simulink model "HANcoder_E407_TTA_CombineModel"  (R2022b)
settings: Solver=FixedStepDiscrete  StartTime=0.0  StopTime=1  FixedStep=0.001  RelTol=1e-3
PreLoadFcn:
  | librarySetup
  | eval([bdroot,'_startup']) %Calling [modelName]_startup.m
values from neighbouring files (symbols this model uses):
  ClockOn = Simulink.Parameter    [HANcoder_E407_TTA_Chris_startup.m]    (also in HANcoder_E407_TTA_CombineModel_Membership_2022a_startup.m; HANcoder_E407_TTA_CombineModel_Membership_startup.m; HANcoder_E407_TTA_CombineModel_V2_startup.m; HANcoder_E407_TTA_CombineModel_startup.m)
  controlWidth = Simulink.Parameter    [HANcoder_E407_TTA_CombineModel_Membership_2022a_startup.m]    (also in HANcoder_E407_TTA_CombineModel_Membership_startup.m; HANcoder_E407_TTA_CombineModel_V2_startup.m; HANcoder_E407_TTA_CombineModel_startup.m)
  desiredAngle = Simulink.Parameter    [HANcoder_E407_TTA_CombineModel_Membership_2022a_startup.m]    (also in HANcoder_E407_TTA_CombineModel_Membership_startup.m; HANcoder_E407_TTA_CombineModel_V2_startup.m; HANcoder_E407_TTA_CombineModel_startup.m)
  frequency_IRQ = 1000    [HANcoder_E407_TTA_Chris_startup.m]    (also in HANcoder_E407_TTA_CombineModel_Membership_2022a_startup.m; HANcoder_E407_TTA_CombineModel_Membership_startup.m; HANcoder_E407_TTA_CombineModel_V2_startup.m; HANcoder_E407_TTA_CombineModel_startup.m)
  intVal = Simulink.Parameter    [HANcoder_E407_TTA_CombineModel_Membership_2022a_startup.m]    (also in HANcoder_E407_TTA_CombineModel_Membership_startup.m; HANcoder_E407_TTA_CombineModel_V2_startup.m; HANcoder_E407_TTA_CombineModel_startup.m)
  L0b = 1    [HANcoder_E407_KinematicAngleControl_startup.m]    (also in HANcoder_E407_TTA_CombineModel_Membership_2022a_startup.m; HANcoder_E407_TTA_CombineModel_Membership_startup.m; HANcoder_E407_TTA_CombineModel_V2_startup.m; HANcoder_E407_TTA_CombineModel_startup.m)
  L0F = 3    [HANcoder_E407_KinematicAngleControl_startup.m]    (also in HANcoder_E407_TTA_CombineModel_Membership_2022a_startup.m; HANcoder_E407_TTA_CombineModel_Membership_startup.m; HANcoder_E407_TTA_CombineModel_V2_startup.m; HANcoder_E407_TTA_CombineModel_startup.m)
  L1F = 4    [HANcoder_E407_KinematicAngleControl_startup.m]    (also in HANcoder_E407_TTA_CombineModel_Membership_2022a_startup.m; HANcoder_E407_TTA_CombineModel_Membership_startup.m; HANcoder_E407_TTA_CombineModel_V2_startup.m; HANcoder_E407_TTA_CombineModel_startup.m)
  matrixRows = Simulink.Parameter    [HANcoder_E407_TTA_Chris_startup.m]    (also in HANcoder_E407_TTA_CombineModel_Membership_2022a_startup.m; HANcoder_E407_TTA_CombineModel_Membership_startup.m; HANcoder_E407_TTA_CombineModel_V2_startup.m; HANcoder_E407_TTA_CombineModel_startup.m)
  MMBS1_ID = Simulink.Parameter    [HANcoder_E407_TTA_Chris_startup.m]    (also in HANcoder_E407_TTA_CombineModel_Membership_2022a_startup.m; HANcoder_E407_TTA_CombineModel_Membership_startup.m; HANcoder_E407_TTA_CombineModel_V2_startup.m; HANcoder_E407_TTA_CombineModel_startup.m)
  propVal = Simulink.Parameter    [HANcoder_E407_TTA_CombineModel_Membership_2022a_startup.m]    (also in HANcoder_E407_TTA_CombineModel_Membership_startup.m; HANcoder_E407_TTA_CombineModel_V2_startup.m; HANcoder_E407_TTA_CombineModel_startup.m)
  ResetPosition = Simulink.Parameter    [HANcoder_E407_TTA_CombineModel_Membership_2022a_startup.m]    (also in HANcoder_E407_TTA_CombineModel_V2_startup.m)
  slotTime = Simulink.Parameter    [HANcoder_E407_TTA_Chris_startup.m]    (also in HANcoder_E407_TTA_CombineModel_Membership_2022a_startup.m; HANcoder_E407_TTA_CombineModel_Membership_startup.m; HANcoder_E407_TTA_CombineModel_V2_startup.m; HANcoder_E407_TTA_CombineModel_startup.m)
  SSTM1_ID = Simulink.Parameter    [HANcoder_E407_TTA_Chris_startup.m]    (also in HANcoder_E407_TTA_CombineModel_Membership_2022a_startup.m; HANcoder_E407_TTA_CombineModel_Membership_startup.m; HANcoder_E407_TTA_CombineModel_V2_startup.m; HANcoder_E407_TTA_CombineModel_startup.m)
  SYNC1_ID = Simulink.Parameter    [HANcoder_E407_TTA_Chris_startup.m]    (also in HANcoder_E407_TTA_CombineModel_Membership_2022a_startup.m; HANcoder_E407_TTA_CombineModel_Membership_startup.m; HANcoder_E407_TTA_CombineModel_V2_startup.m; HANcoder_E407_TTA_CombineModel_startup.m)
  TRCK1_ID1 = Simulink.Parameter    [HANcoder_E407_TTA_Chris_startup.m]    (also in HANcoder_E407_TTA_CombineModel_Membership_2022a_startup.m; HANcoder_E407_TTA_CombineModel_Membership_startup.m; HANcoder_E407_TTA_CombineModel_V2_startup.m; HANcoder_E407_TTA_CombineModel_startup.m)
  TRCK1_ID2 = Simulink.Parameter    [HANcoder_E407_TTA_Chris_startup.m]    (also in HANcoder_E407_TTA_CombineModel_Membership_2022a_startup.m; HANcoder_E407_TTA_CombineModel_Membership_startup.m; HANcoder_E407_TTA_CombineModel_V2_startup.m; HANcoder_E407_TTA_CombineModel_startup.m)
  TRCK1_ID3 = Simulink.Parameter    [HANcoder_E407_TTA_Chris_startup.m]    (also in HANcoder_E407_TTA_CombineModel_Membership_2022a_startup.m; HANcoder_E407_TTA_CombineModel_Membership_startup.m; HANcoder_E407_TTA_CombineModel_V2_startup.m; HANcoder_E407_TTA_CombineModel_startup.m)
  TRLS1_ID4 = Simulink.Parameter    [HANcoder_E407_TTA_Chris_startup.m]    (also in HANcoder_E407_TTA_CombineModel_Membership_2022a_startup.m; HANcoder_E407_TTA_CombineModel_Membership_startup.m; HANcoder_E407_TTA_CombineModel_V2_startup.m; HANcoder_E407_TTA_CombineModel_startup.m)
  TRLS1_ID5 = Simulink.Parameter    [HANcoder_E407_TTA_Chris_startup.m]    (also in HANcoder_E407_TTA_CombineModel_Membership_2022a_startup.m; HANcoder_E407_TTA_CombineModel_Membership_startup.m; HANcoder_E407_TTA_CombineModel_V2_startup.m; HANcoder_E407_TTA_CombineModel_startup.m)
  V2 = 1.3889    [HANcoder_E407_KinematicAngleControl_startup.m]    (also in HANcoder_E407_TTA_CombineModel_Membership_2022a_startup.m = 0.5; HANcoder_E407_TTA_CombineModel_Membership_startup.m = 0.5; HANcoder_E407_TTA_CombineModel_V2_startup.m = 0.5; HANcoder_E407_TTA_CombineModel_startup.m = 0.5)
undefined symbols (not defined in the file or in its folder): A2, A3, A4, CON2, CON3, CON4, D10, D4, D5
libraries: hdlsllib x95, HANcoder_STM32_Target x23, simulink_extras x4, dspstat3 x3, simulink x2, slpidlib x1
(part 1 of 5)
settings Model: Creator=Jason van Kolfschoten  LastModifiedBy=Admin.cvanderspek
settings SolverCC: AlgebraicLoopSolver=TrustRegion  PositivePriorityOrder=on
settings DataIOCC: LimitDataPoints=on  SaveFormat=Array  SignalLoggingSaveFormat=ModelDataLogs  SaveOutput=off  SignalLogging=off  DSMLogging=off  SaveTime=off  ReturnWorkspaceOutputs=off
settings OptimizationCC: BlockReduction=off  DefaultParameterBehavior=Inlined  DefaultUnderspecifiedDataType=single  InlineInvariantSignals=on  ExpressionDepthLimit=2147483647  StateBitsets=on  DataBitsets=on  ZeroExternalMemoryAtStartup=off  ZeroInternalMemoryAtStartup=off  InitFltsAndDblsToZero=on  NoFixptDivByZeroProtection=on  EfficientFloat2IntCast=on  LifeSpan=inf  EfficientTunableParamExpr=on
settings DebuggingCC: SaveWithDisabledLinksMsg=none  SaveWithParameterizedLinksMsg=none  CheckSSInitialOutputMsg=off  UnderspecifiedInitializationDetection=Classic  MergeDetectMultiDrivingBlocksExec=none  SignalResolutionControl=TryResolveAll  SolverPrmCheckMsg=warning  InheritedTsInSrcMsg=none  MultiTaskDSMMsg=warning  MultiTaskCondExecSysMsg=none  ParameterPrecisionLossMsg=none  FcnCallInpInsideContextMsg=warning  UnconnectedInputMsg=warning  UnconnectedOutputMsg=warning  UnconnectedLineMsg=warning  StateNameClashWarn=warning  SFUnexpectedBacktrackingDiag=warning  SFNoUnconditionalDefaultTransitionDiag=warning  SFExecutionAtInitializationDiag=none  SFMachineParentedDataDiag=warning  ArithmeticOperatorsInVariantConditions=warning
settings HardwareCC: ProdBitPerPointer=32  ProdBitPerSizeT=32  ProdBitPerPtrDiffT=32  ProdLargestAtomicInteger=Long  ProdLargestAtomicFloat=Double  ProdWordSize=32  ProdHWDeviceType=ARM Compatible->ARM Cortex  TargetEndianess=LittleEndian  TargetHWDeviceType=Infineon->TriCore
settings ModelReferenceCC: PropagateSignalLabelsOutOfModel=off
settings SFSimCC: SimUseLocalCustomCode=off  MATLABDynamicMemAlloc=off  CustomCodeUndefinedFunction=UseInterfaceOnly
settings RTWCC: Description=Real-Time Workshop Embedded Coder (no auto configuration)  SystemTargetFile=ert.tlc  MakeCommand=make_rtw SHELL= HANcoder_PORTABLE=1 HANcoder_BOOTLOADER=1  TemplateMakefile=STM32_E407_gcc.tmf  RTWUseLocalCustomCode=off
settings CodeAppCC: ForceParamTrailComments=on  IgnoreCustomStorageClasses=off  SimulinkDataObjDesc=on  CustomSymbolStrGlobalVar=rt$N$M  CustomSymbolStrType=$N$M  CustomSymbolStrFcn=$N$M$F  CustomSymbolStrMacro=$N$M  InsertBlockDesc=on  StateflowObjectComments=on  InternalIdentifier=Classic
settings ERTTargetCC: TargetFcnLib=ansi_tfl_tmw.mat  MultiwordLength=2048  IncludeMdlTerminateFcn=off  SuppressErrorStatus=on  SupportNonFinite=off  GenerateASAP2=on  InlinedParameterPlacement=NonHierarchical  ERTCustomFileTemplate=example_file_process.tlc  ConvertIfToSwitch=off  SuppressUnreachableDefaultCases=off
settings ConfigComp: CovMetricSettings=dw  CovSaveCumulativeToWorkspaceVar=on  CovSaveSingleToWorkspaceVar=on  CovExternalEMLEnable=off  CovSFcnEnable=off  DVMaxProcessTime=600  DVAutomaticStubbing=off  DVModelCoverageObjectives=MCDC  DVMaxTestCaseSteps=500  DVTestSuiteOptimization=CombinedObjectives  DVDetectActiveLogic=on  DVSaveHarnessModel=on  DVHarnessSource=Signal Editor

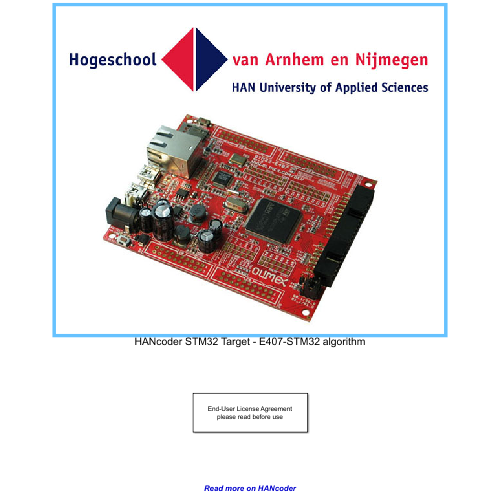
[thumbnail: Simulink's stored preview of the top-level diagram]
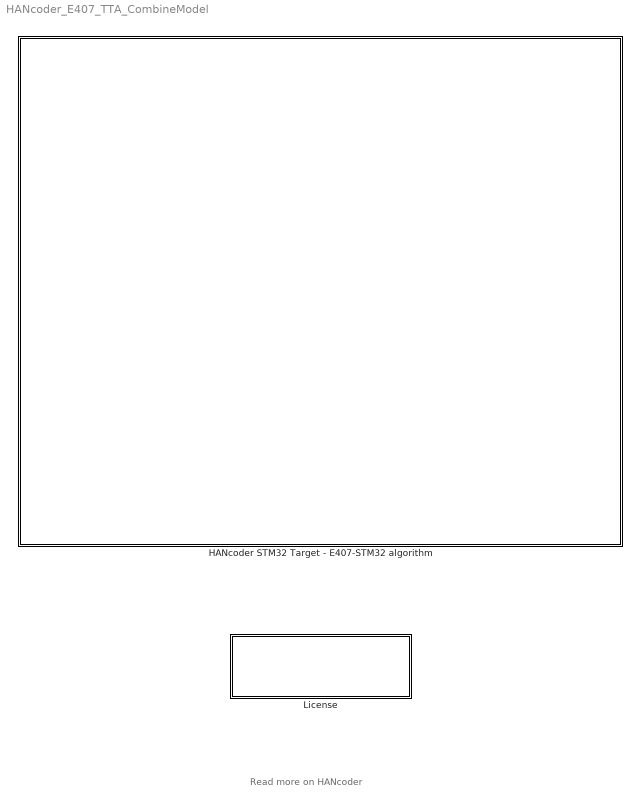
== system HANcoder_E407_TTA_CombineModel ==
  note: Read more on HANcoder
  HANcoder STM32 Target - E407-STM32 algorithm : Subsystem  mask(TopLevelSubsystem){}
      settings: CopyFcn=HANcoderChecks('Copy');  NameChangeFcn=HANcoderChecks('NameChangeE407');  MoveFcn=HANcoderChecks('MoveE407');
      mask Display: image(imread('STM32_E407_HAN.jpg'))
  License : Subsystem  mask(License){}
      settings: NameChangeFcn=HANcoderChecks('NameChangeLicenseBlock');  OpenFcn=winopen('License.pdf')  MoveFcn=HANcoderChecks('MoveLicenseBlock');
      mask Display: disp(['End-User License Agreement\n','please read before use']);

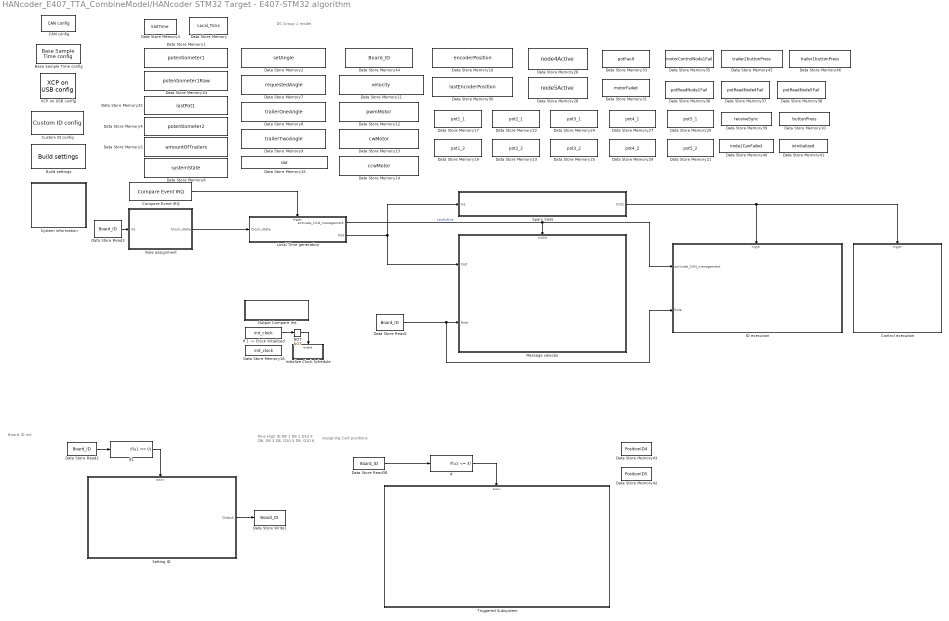
== system HANcoder_E407_TTA_CombineModel/HANcoder STM32 Target - E407-STM32 algorithm ==
  note: DS Group 1 model
  note: Assigning Cart positions
  note: Board ID init
  note: Pins High      		ID
      | D8                 		1
      | D9				2
      | D10				4
      | D8, D9			3
      | D8, D10			5
      | D9, D10			6
  Base Sample Time config : HANcoder_STM32_Target/STM32-E407/System Config/Base Sample Time config  Tag=HANcoder_TARGET_STM32_E407  Description=HANcoder Target STM32-E407 blockset version 1.0  baseSampleTime=1  extraStack=100
      settings: SourceProductName=HANcoder STM32 Target
  Build settings : HANcoder_STM32_Target/STM32-E407/System Config/Build settings  Tag=HANcoder_TARGET_STM32_E407  AutoASAP2add=on  AutoFlash=USB
      settings: SourceProductName=HANcoder STM32 Target
  CAN config : HANcoder_STM32_Target/STM32-E407/System Config/CAN config  Tag=HANcoder_TARGET_STM32_E407  txBufSize=64  evBufSize=8  canBus1=on  baudRate1=1000  rxMask1=hex2dec('00000000')  rxCode1=hex2dec('00000000')  rxMode1=Receive only 11-bit message identifiers  canBus2=off  baudRate2=250  rxMask2=hex2dec('00000000')  rxCode2=hex2dec('00000000')  rxMode2=Receive only 11-bit message identifiers
      settings: SourceProductName=HANcoder STM32 Target
  Compare Event IRQ : HANcoder_STM32_Target/STM32-E407/Timer Outputs/Compare Event IRQ  Tag=HANcoder_TARGET_STM32_E407  Priority=20  pin=TIM4 - CON PD - 15 - 5V Tolerant
      settings: SourceProductName=HANcoder STM32 Target
  Control execution : Subsystem
  Custom ID config : HANcoder_STM32_Target/STM32-E407/System Config/Custom ID config  Tag=HANcoder_TARGET_STM32_E407  softID=softwareID  softNUM=1
      settings: SourceProductName=HANcoder STM32 Target
  Data Store Memory : DataStoreMemory  DataStoreName=Local_Ticks  WriteAfterWriteMsg=warning  ShowAdditionalParam=off  OutDataTypeStr=uint8
  Data Store Memory1 : DataStoreMemory  DataStoreName=potentiometer1  WriteAfterWriteMsg=warning  ShowAdditionalParam=off  OutDataTypeStr=uint16
  Data Store Memory10 : DataStoreMemory  DataStoreName=buttonPress  WriteAfterWriteMsg=warning  ShowAdditionalParam=off  OutDataTypeStr=uint8
  Data Store Memory11 : DataStoreMemory  DataStoreName=velocity  WriteAfterWriteMsg=warning  ShowAdditionalParam=off  OutDataTypeStr=uint8
  Data Store Memory12 : DataStoreMemory  DataStoreName=pwmMotor  WriteAfterWriteMsg=warning  ShowAdditionalParam=off  OutDataTypeStr=uint16
  Data Store Memory13 : DataStoreMemory  DataStoreName=cwMotor  WriteAfterWriteMsg=warning  ShowAdditionalParam=off
  Data Store Memory14 : DataStoreMemory  DataStoreName=ccwMotor  WriteAfterWriteMsg=warning  ShowAdditionalParam=off
  Data Store Memory15 : DataStoreMemory  DataStoreName=slot  WriteAfterWriteMsg=warning  ShowAdditionalParam=off  OutDataTypeStr=uint8
  Data Store Memory16 : DataStoreMemory  DataStoreName=encoderPosition  WriteAfterWriteMsg=warning  ShowAdditionalParam=off  OutDataTypeStr=int32
  Data Store Memory17 : DataStoreMemory  DataStoreName=pot1_1  WriteAfterWriteMsg=warning  ShowAdditionalParam=off  OutDataTypeStr=uint16
  Data Store Memory18 : DataStoreMemory  Priority=1  DataStoreName=init_clock  ReadBeforeWriteMsg=warning  WriteAfterWriteMsg=warning  WriteAfterReadMsg=warning  ShowAdditionalParam=off
  Data Store Memory19 : DataStoreMemory  DataStoreName=pot1_2  WriteAfterWriteMsg=warning  ShowAdditionalParam=off  OutDataTypeStr=uint16
  Data Store Memory2 : DataStoreMemory  DataStoreName=setAngle  WriteAfterWriteMsg=warning  ShowAdditionalParam=off
  Data Store Memory20 : DataStoreMemory  DataStoreName=pot5_1  WriteAfterWriteMsg=warning  ShowAdditionalParam=off  OutDataTypeStr=uint16
  Data Store Memory21 : DataStoreMemory  DataStoreName=pot5_2  WriteAfterWriteMsg=warning  ShowAdditionalParam=off  OutDataTypeStr=uint16
  Data Store Memory22 : DataStoreMemory  DataStoreName=pot2_1  WriteAfterWriteMsg=warning  ShowAdditionalParam=off  OutDataTypeStr=uint16
  Data Store Memory23 : DataStoreMemory  DataStoreName=pot2_2  WriteAfterWriteMsg=warning  ShowAdditionalParam=off  OutDataTypeStr=uint16
  Data Store Memory24 : DataStoreMemory  DataStoreName=pot3_1  WriteAfterWriteMsg=warning  ShowAdditionalParam=off  OutDataTypeStr=uint16
  Data Store Memory25 : DataStoreMemory  DataStoreName=pot3_2  WriteAfterWriteMsg=warning  ShowAdditionalParam=off  OutDataTypeStr=uint16
  Data Store Memory26 : DataStoreMemory  DataStoreName=node4Active  WriteAfterWriteMsg=warning  ShowAdditionalParam=off  OutDataTypeStr=boolean
  Data Store Memory27 : DataStoreMemory  DataStoreName=pot4_1  WriteAfterWriteMsg=warning  ShowAdditionalParam=off  OutDataTypeStr=uint16
  Data Store Memory28 : DataStoreMemory  DataStoreName=node5Active  WriteAfterWriteMsg=warning  ShowAdditionalParam=off  OutDataTypeStr=boolean
  Data Store Memory29 : DataStoreMemory  DataStoreName=pot4_2  WriteAfterWriteMsg=warning  ShowAdditionalParam=off  OutDataTypeStr=uint16
  Data Store Memory3 : DataStoreMemory  DataStoreName=SlotTime  WriteAfterWriteMsg=warning  ShowAdditionalParam=off  OutDataTypeStr=uint8
  Data Store Memory30 : DataStoreMemory  DataStoreName=lastEncoderPosition  WriteAfterWriteMsg=warning  ShowAdditionalParam=off  OutDataTypeStr=int32
  Data Store Memory31 : DataStoreMemory  DataStoreName=motorFailed  WriteAfterWriteMsg=warning  ShowAdditionalParam=off  OutDataTypeStr=boolean
  Data Store Memory32 : DataStoreMemory  DataStoreName=lastPot1  WriteAfterWriteMsg=warning  ShowAdditionalParam=off  OutDataTypeStr=uint16
  Data Store Memory33 : DataStoreMemory  DataStoreName=potFault  WriteAfterWriteMsg=warning  ShowAdditionalParam=off  OutDataTypeStr=boolean
  Data Store Memory34 : DataStoreMemory  DataStoreName=potentiometer1Raw  WriteAfterWriteMsg=warning  ShowAdditionalParam=off  OutDataTypeStr=uint16
  Data Store Memory35 : DataStoreMemory  DataStoreName=motorControlNode1Fail  WriteAfterWriteMsg=warning  ShowAdditionalParam=off  OutDataTypeStr=boolean
  Data Store Memory36 : DataStoreMemory  DataStoreName=potReadNode1Fail  WriteAfterWriteMsg=warning  ShowAdditionalParam=off  OutDataTypeStr=boolean
  Data Store Memory37 : DataStoreMemory  DataStoreName=potReadNode4Fail  WriteAfterWriteMsg=warning  ShowAdditionalParam=off  OutDataTypeStr=boolean
  Data Store Memory38 : DataStoreMemory  DataStoreName=potReadNode5Fail  WriteAfterWriteMsg=warning  ShowAdditionalParam=off  OutDataTypeStr=boolean
  Data Store Memory39 : DataStoreMemory  DataStoreName=receiveSync  WriteAfterWriteMsg=warning  ShowAdditionalParam=off  OutDataTypeStr=boolean
  Data Store Memory4 : DataStoreMemory  DataStoreName=potentiometer2  WriteAfterWriteMsg=warning  ShowAdditionalParam=off  OutDataTypeStr=uint16
  Data Store Memory40 : DataStoreMemory  DataStoreName=node1CanFailed  WriteAfterWriteMsg=warning  ShowAdditionalParam=off  OutDataTypeStr=boolean
  Data Store Memory41 : DataStoreMemory  DataStoreName=ioInitialized  WriteAfterWriteMsg=warning  ShowAdditionalParam=off
  Data Store Memory42 : DataStoreMemory  DataStoreName=PositionID5  WriteAfterWriteMsg=warning  ShowAdditionalParam=off  OutDataTypeStr=uint8
  Data Store Memory43 : DataStoreMemory  DataStoreName=PositionID4  WriteAfterWriteMsg=warning  ShowAdditionalParam=off  OutDataTypeStr=uint8
  Data Store Memory44 : DataStoreMemory  Priority=10  DataStoreName=Board_ID  ReadBeforeWriteMsg=warning  WriteAfterWriteMsg=warning  WriteAfterReadMsg=warning  ShowAdditionalParam=off  OutDataTypeStr=uint8
  Data Store Memory45 : DataStoreMemory  DataStoreName=trailer2buttonPress  WriteAfterWriteMsg=warning  ShowAdditionalParam=off
  Data Store Memory46 : DataStoreMemory  DataStoreName=trailer1buttonPress  WriteAfterWriteMsg=warning  ShowAdditionalParam=off
  Data Store Memory5 : DataStoreMemory  DataStoreName=amountOfTrailers  WriteAfterWriteMsg=warning  ShowAdditionalParam=off
  Data Store Memory6 : DataStoreMemory  DataStoreName=systemState  WriteAfterWriteMsg=warning  ShowAdditionalParam=off
  Data Store Memory7 : DataStoreMemory  DataStoreName=requestedAngle  WriteAfterWriteMsg=warning  ShowAdditionalParam=off
  Data Store Memory8 : DataStoreMemory  DataStoreName=trailerOneAngle  WriteAfterWriteMsg=warning  ShowAdditionalParam=off  OutDataTypeStr=uint16
  Data Store Memory9 : DataStoreMemory  DataStoreName=trailerTwoAngle  WriteAfterWriteMsg=warning  ShowAdditionalParam=off  OutDataTypeStr=uint16
  Data Store Read1 : DataStoreRead  DataStoreName=Board_ID  IndexOptions=Index vector (dialog)  Indices=1  OutputSizes=1
  Data Store Read2 : DataStoreRead  Priority=10  DataStoreName=Board_ID  IndexOptions=Index vector (dialog)  Indices=1  OutputSizes=1
  Data Store Read3 : DataStoreRead  DataStoreName=Board_ID  IndexOptions=Index vector (dialog)  Indices=1  OutputSizes=1
  Data Store Read38 : DataStoreRead  DataStoreName=Board_ID  IndexOptions=Index vector (dialog)  Indices=1  OutputSizes=1
  Data Store Write1 : DataStoreWrite  Priority=13  DataStoreName=Board_ID  IndexOptions=Index vector (dialog)  Indices=1  OutputSizes=1
  IO execution : Subsystem
  If : If  IfExpression=u1 <= 3  ShowElse=off
  "If 1 -> Clock initialized " : DataStoreRead  Priority=2  DataStoreName=init_clock  IndexOptions=Index vector (dialog)  Indices=1  OutputSizes=1
  If1 : If  Priority=11  IfExpression=u1 == 0  ShowElse=off
  Initialize Clock Schedule : Subsystem  Priority=4  TreatAsAtomicUnit=on
  Local Time generation : Subsystem  TreatAsAtomicUnit=on
  Message selector : Subsystem  Description=Truck 1  TreatAsAtomicUnit=on
  NOT : Logic  Priority=3  Operator=NOT  IconShape=distinctive  AllPortsSameDT=off  OutDataTypeStr=boolean
  Output Compare Init : Subsystem  Tag=HANcoder_TARGET_STM32_E407  AncestorBlock=HANcoder_STM32_Target/STM32-E407/Timer Outputs/Output Compare Init  mask(Output Compare Init){moduleID=TIM4 - CON PD - 15 & 16 &n/a & n/a, frequency=1000000, enableIRQoutput=off}
      mask prompts: moduleID "Timer module"; frequency "Frequency (free running counter) [Hz]"; enableIRQoutput "Enable IRQ output"
      mask help:
      | Function
      | ========
      | Initializes the timer module to allow output compare functionality on the
      | module's channels.
      |
      | Parameters
      | ==========
      | Timer Module:
      |   Selects the timer module.
      |
      | Frequency:
      |   Frequency at which the 16-bit free running counter counts.
      |
      | Enable IRQ output
      |   Controls whether or not the IRQ output is available.
      |
      | Outport
      | =======
      | IRQ
      |   Allows connection of a function call subsystem for the free running
      |   counter overflow event.
      mask init:
      | moduleIDInfoStr = sfcn_timeout_init_mcb(2, moduleID, frequency, enableIRQoutput);
      settings: LibrarySourceBlock=HANcoder_STM32_Target/STM32-E407/Timer Outputs/Output Compare Init  CopyFcn=sfcn_timeout_init_chk();  MoveFcn=drawLogos
      mask Help: web('sfcn_timeout_init.html');
      mask TypeOptions moduleID: TIM1 - CON PE - 12 & 14 & 16 & 17 | TIM2 - CON4 - D13 & n/a & n/a & n/a | TIM3 - CON4 - D12 & D11 & n/a & n/a | TIM4 - CON PD - 15 & 16 &n/a & n/a | TIM8 - UEXT - 3 & 4 & n/a & n/a | TIM9 - CON3 - D4 & D5 or PE - 8 & 9 | TIM10 - CON2 - A1 or CON PF - 9 | TIM11 - CON2 - A2 or CON PF - 10 | TIM13 - CON2 - A3 or CON PF - 11 | TIM14 - CON2 - A4 or CON PF - 12
      mask Callback moduleID: sfcn_timeout_init_chk();
      mask Display: fprintf('Output Compare Init\n%s', moduleIDInfoStr);patch([135 141 141],[8 14 2],[1 0 0]);patch([143 143 149],[14 2 8],[0 0 0.35]);
  Role assignment : Subsystem
  Setting ID : Subsystem
  Spars Slots : Subsystem
  System information : Subsystem
  Triggered Subsystem : Subsystem  TreatAsAtomicUnit=on
  XCP on USB config : HANcoder_STM32_Target/STM32-E407/System Config/XCP on USB config  Tag=HANcoder_TARGET_STM32_E407
      settings: SourceProductName=HANcoder STM32 Target
  wires:
  Compare Event IRQ/1 -> Local Time generation/Trigger
  NOT/1 -> Initialize Clock Schedule/Enable
  "If 1 -> Clock initialized "/1 -> NOT/1
  Role assignment/1(Clock_State) -> Local Time generation/1(Clock_State)
  Local Time generation/1(activate_CAN_management) -> Message selector/Enable, IO execution/1(activate_CAN_management)  "canActive"
  Data Store Read1/1 -> IO execution/2(Role), Message selector/2(Role)
  Local Time generation/2(Slot) -> Spars Slots/1(In1), Message selector/1(Slot)
  Spars Slots/1(Out1) -> IO execution/Trigger, Control execution/Trigger
  If/1 -> Triggered Subsystem/Action
  Data Store Read38/1 -> If/1
  Data Store Read2/1 -> If1/1
  Setting ID/1(Output) -> Data Store Write1/1
  If1/1 -> Setting ID/Action
  Data Store Read3/1 -> Role assignment/1(In1)

== system HANcoder_E407_TTA_CombineModel/License ==

== system HANcoder_E407_TTA_CombineModel/HANcoder STM32 Target - E407-STM32 algorithm/Control execution ==
  Trigger : TriggerPort  VariantControl=(inherit)  PortDimensions=1
  Constant : Constant  Value=V2
  Constant1 : Constant  Value=0
  Control Algorithm : Subsystem
  Data Store Read : DataStoreRead  DataStoreName=requestedAngle  IndexOptions=Index vector (dialog)  Indices=1  OutputSizes=1
  Data Store Read1 : DataStoreRead  DataStoreName=trailerOneAngle  IndexOptions=Index vector (dialog)  Indices=1  OutputSizes=1
  Data Store Read2 : DataStoreRead  DataStoreName=trailerTwoAngle  IndexOptions=Index vector (dialog)  Indices=1  OutputSizes=1
  Data Store Write : DataStoreWrite  DataStoreName=pwmMotor  IndexOptions=Index vector (dialog)  Indices=1  OutputSizes=1
  Data Store Write1 : DataStoreWrite  DataStoreName=cwMotor  IndexOptions=Index vector (dialog)  Indices=1  OutputSizes=1
  Data Store Write8 : DataStoreWrite  DataStoreName=ccwMotor  IndexOptions=Index vector (dialog)  Indices=1  OutputSizes=1
  Kinematic Algorithm : Subsystem
  wires:
  Constant/1 -> Kinematic Algorithm/2(V2)
  Kinematic Algorithm/1(Delta12K) -> Control Algorithm/1(Kinematic output)  "delta12K"
  Data Store Read1/1 -> Kinematic Algorithm/4(YawTrailer1Angle)  "t1Angle"
  Data Store Read/1 -> Kinematic Algorithm/1(DeltaC)  "reqAngle"
  Constant1/1 -> Kinematic Algorithm/3(YawTractorAngle)
  Data Store Read2/1 -> Kinematic Algorithm/5(YawTrailer2Angle)  "t2Angle"
  Control Algorithm/1(Motor speed) -> Data Store Write/1
  Control Algorithm/2(CW direction) -> Data Store Write1/1
  Control Algorithm/3(CCW direction) -> Data Store Write8/1

== system HANcoder_E407_TTA_CombineModel/HANcoder STM32 Target - E407-STM32 algorithm/IO execution ==
  activate_CAN_management : Inport
  Role : Inport  Port=2
  Trigger : TriggerPort  VariantControl=(inherit)  PortDimensions=1
  Data Store Read : DataStoreRead  DataStoreName=pwmMotor  IndexOptions=Index vector (dialog)  Indices=1  OutputSizes=1
  Data Store Read1 : DataStoreRead  DataStoreName=cwMotor  IndexOptions=Index vector (dialog)  Indices=1  OutputSizes=1
  Data Store Read3 : DataStoreRead  DataStoreName=ccwMotor  IndexOptions=Index vector (dialog)  Indices=1  OutputSizes=1
  Inputs : Subsystem
  Outputs : Subsystem
  Voting : Subsystem
  wires:
  Data Store Read/1 -> Outputs/1(PWM mospeed)
  Data Store Read1/1 -> Outputs/2(CW signal)
  Data Store Read3/1 -> Outputs/3(CCW signal)
  Role/1 -> Outputs/4(Role), Voting/1(Role)
  activate_CAN_management/1 -> Outputs/5(activate_CAN_management)

== system HANcoder_E407_TTA_CombineModel/HANcoder STM32 Target - E407-STM32 algorithm/Initialize Clock Schedule ==
  Enable : EnablePort
  Constant : Constant  OutDataTypeStr=uint16
  Constant1 : Constant  Value=3  OutDataTypeStr=uint8
  Constant2 : Constant
  Data Store Write : DataStoreWrite  DataStoreName=init_clock  IndexOptions=Index vector (dialog)  Indices=1  OutputSizes=1
  Schedule Compare Event : HANcoder_STM32_Target/STM32-E407/Timer Outputs/Schedule Compare Event  Tag=HANcoder_TARGET_STM32_E407  pin=TIM4 - CON PD - 15 - 5V Tolerant  tsamp=-1
      settings: SourceProductName=HANcoder STM32 Target
  wires:
  Constant/1 -> Schedule Compare Event/1
  Constant1/1 -> Schedule Compare Event/2
  Constant2/1 -> Data Store Write/1

== system HANcoder_E407_TTA_CombineModel/HANcoder STM32 Target - E407-STM32 algorithm/Local Time generation ==
  note: Reschedule IRQ activation
  note: Cycle update
  Clock_State : Inport
  function : TriggerPort  TriggerType=function-call  VariantControl=Variant
  Cast : DataTypeConversion  OutDataTypeStr=uint16  SaturateOnIntegerOverflow=off  RndMeth=Floor
  Constant : Constant  Value=frequency_IRQ  OutDataTypeStr=uint16
  Constant1 : Constant  Value=3  OutDataTypeStr=uint8
  Constant2 : Constant  OutDataTypeStr=uint8
  Data Store Read : DataStoreRead  DataStoreName=Local_Ticks  IndexOptions=Index vector (dialog)  Indices=1  OutputSizes=1
  Data Store Read1 : DataStoreRead  DataStoreName=Local_Ticks  IndexOptions=Index vector (dialog)  Indices=1  OutputSizes=1
  Data Store Read2 : DataStoreRead  DataStoreName=Local_Ticks  IndexOptions=Index vector (dialog)  Indices=1  OutputSizes=1
  Data Store Read3 : DataStoreRead  DataStoreName=SlotTime  IndexOptions=Index vector (dialog)  Indices=1  OutputSizes=1
  Data Store Write : DataStoreWrite  DataStoreName=Local_Ticks  IndexOptions=Index vector (dialog)  Indices=1  OutputSizes=1
  Enabled Subsystem : Subsystem  TreatAsAtomicUnit=on
  Equal : RelationalOperator  OutDataTypeStr=boolean  RndMeth=Simplest  InputSameDT=off
  Get Last Event Counter : HANcoder_STM32_Target/STM32-E407/Timer Outputs/Get Last Event Counter  Tag=HANcoder_TARGET_STM32_E407  pin=TIM4 - CON PD - 15 - 5V Tolerant  tsamp=-1
      settings: SourceProductName=HANcoder STM32 Target
  Schedule Compare Event1 : HANcoder_STM32_Target/STM32-E407/Timer Outputs/Schedule Compare Event  Tag=HANcoder_TARGET_STM32_E407  pin=TIM4 - CON PD - 15 - 5V Tolerant  tsamp=-1
      settings: SourceProductName=HANcoder STM32 Target
  Sum : Sum
  Sum1 : Sum  AccumDataTypeStr=uint8
  Switch : Switch  Criteria=u2 > Threshold  OutDataTypeStr=uint8  SaturateOnIntegerOverflow=off  InputSameDT=off
  activate_CAN_management : Outport  VectorParamsAs1DForOutWhenUnconnected=off
  Slot : Outport  Port=2
  wires:
  Get Last Event Counter/1 -> Sum/1
  Constant/1 -> Sum/2
  Sum/1 -> Schedule Compare Event1/1
  Constant1/1 -> Schedule Compare Event1/2
  Data Store Read1/1 -> Switch/3
  Data Store Read/1 -> Sum1/1
  Constant2/1 -> Sum1/2
  Switch/1 -> Data Store Write/1  "local_ticks_interrupt"
  Sum1/1 -> Switch/1
  Clock_State/1 -> activate_CAN_management/1, Switch/2
  Data Store Read2/1 -> Equal/1
  Enabled Subsystem/1(Out1) -> Slot/1
  Equal/1 -> Enabled Subsystem/Trigger
  Data Store Read3/1 -> Cast/1  "setSlotTime"
  Cast/1 -> Equal/2

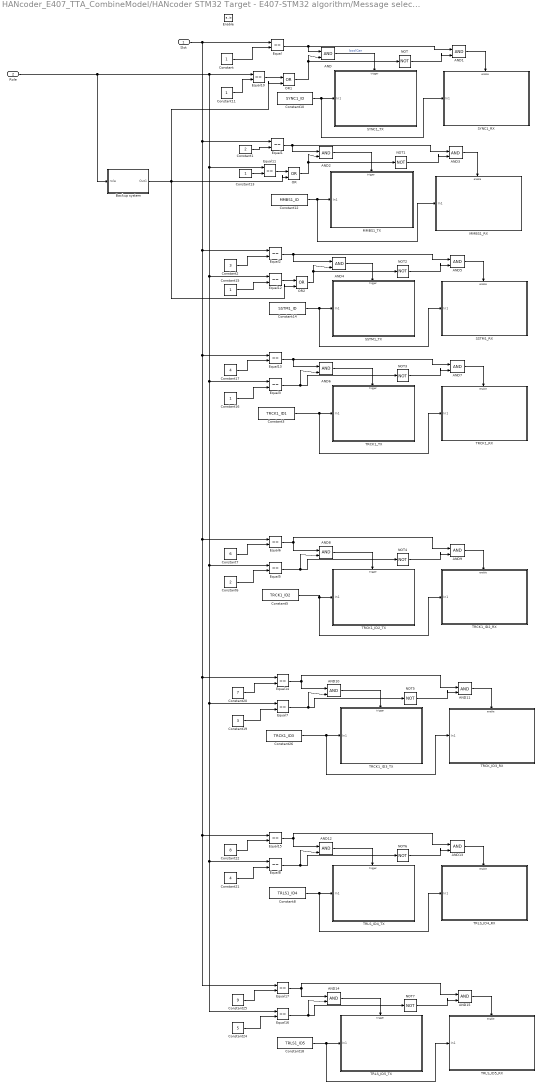
== system HANcoder_E407_TTA_CombineModel/HANcoder STM32 Target - E407-STM32 algorithm/Message selector ==
  Slot : Inport
  Role : Inport  Port=2
  Enable : EnablePort
  AND{,1..15} (16 alike) : Logic  IconShape=distinctive  AllPortsSameDT=off  OutDataTypeStr=boolean
  Backup system : Subsystem
  Constant : Constant  OutDataTypeStr=uint8
  Constant1 : Constant  Value=2
  Constant10 : Constant  Value=SYNC1_ID  OutDataTypeStr=uint32
  Constant11 : Constant  OutDataTypeStr=uint8
  Constant12 : Constant  Value=MMBS1_ID  OutDataTypeStr=uint32
  Constant13 : Constant
  Constant14 : Constant  Value=SSTM1_ID  OutDataTypeStr=uint32
  Constant15 : Constant
  Constant16 : Constant
  Constant17 : Constant  Value=4
  Constant18 : Constant  Value=TRLS1_ID5  OutDataTypeStr=uint32
  Constant19 : Constant  Value=3
  Constant2 : Constant  Value=3
  Constant20 : Constant  Value=7
  Constant21 : Constant  Value=4
  Constant22 : Constant  Value=8
  Constant24 : Constant  Value=5
  Constant25 : Constant  Value=9
  Constant26 : Constant  Value=TRCK1_ID3  OutDataTypeStr=uint32
  Constant3 : Constant  Value=TRCK1_ID1  OutDataTypeStr=uint32
  Constant5 : Constant  Value=TRCK1_ID2  OutDataTypeStr=uint32
  Constant6 : Constant  Value=2
  Constant7 : Constant  Value=6
  Constant8 : Constant  Value=TRLS1_ID4  OutDataTypeStr=uint32
  Equal{,1..3,5..8,10..17} (16 alike) : RelationalOperator  Operator===  OutDataTypeStr=boolean  RndMeth=Simplest  InputSameDT=off
  MMBS1_RX : Subsystem
  MMBS1_TX : Subsystem
  NOT{,1..7} (8 alike) : Logic  Operator=NOT  IconShape=distinctive  AllPortsSameDT=off  OutDataTypeStr=boolean
  OR : Logic  Operator=OR  IconShape=distinctive  AllPortsSameDT=off  OutDataTypeStr=boolean
  OR1 : Logic  Operator=OR  IconShape=distinctive  AllPortsSameDT=off  OutDataTypeStr=boolean
  OR2 : Logic  Operator=OR  IconShape=distinctive  AllPortsSameDT=off  OutDataTypeStr=boolean
  SSTM1_RX : Subsystem
  SSTM1_TX : Subsystem
  SYNC1_RX : Subsystem
  SYNC1_TX : Subsystem
  TRCK1_ID2_RX : Subsystem
  TRCK1_ID2_TX : Subsystem
  TRCK1_ID3_TX : Subsystem
  TRCK1_RX : Subsystem
  TRCK1_TX : Subsystem
  TRCK_ID3_RX : Subsystem
  TRLS_ID4_RX : Subsystem
  TRLS_ID4_TX : Subsystem
  TRLS_ID5_RX : Subsystem
  TRLS_ID5_TX : Subsystem
  wires:
  Constant/1 -> Equal/2
  Constant1/1 -> Equal1/2
  Constant2/1 -> Equal2/2
  Constant10/1 -> SYNC1_RX/1(In1), SYNC1_TX/1(In1)
  AND/1 -> SYNC1_TX/Trigger  "boolCan"
  Equal/1 -> AND/1, AND1/1
  AND1/1 -> SYNC1_RX/Enable
  NOT/1 -> AND1/2
  Constant11/1 -> Equal10/2
  Equal1/1 -> AND3/1, AND2/1
  Constant12/1 -> MMBS1_RX/1(In1), MMBS1_TX/1(In1)
  NOT1/1 -> AND3/2
  AND2/1 -> MMBS1_TX/Trigger
  AND3/1 -> MMBS1_RX/Enable
  NOT2/1 -> AND5/2
  AND4/1 -> SSTM1_TX/Trigger
  Constant14/1 -> SSTM1_RX/1(In1), SSTM1_TX/1(In1)
  AND5/1 -> SSTM1_RX/Enable
  Equal2/1 -> AND5/1, AND4/1
  Constant15/1 -> Equal12/2
  Constant16/1 -> Equal3/2
  Equal13/1 -> AND7/1, AND6/1
  Equal3/1 -> AND6/2, NOT3/1
  AND7/1 -> TRCK1_RX/Enable
  Constant3/1 -> TRCK1_RX/1(In1), TRCK1_TX/1(In1)
  AND6/1 -> TRCK1_TX/Trigger
  NOT3/1 -> AND7/2
  Constant17/1 -> Equal13/2
  Constant6/1 -> Equal5/2
  Equal6/1 -> AND9/1, AND8/1
  Equal5/1 -> AND8/2, NOT4/1
  AND9/1 -> TRCK1_ID2_RX/Enable
  Constant5/1 -> TRCK1_ID2_RX/1(In1), TRCK1_ID2_TX/1(In1)
  AND8/1 -> TRCK1_ID2_TX/Trigger
  NOT4/1 -> AND9/2
  Constant7/1 -> Equal6/2
  Constant19/1 -> Equal7/2
  Equal14/1 -> AND11/1, AND10/1
  Equal7/1 -> AND10/2, NOT5/1
  AND11/1 -> TRCK_ID3_RX/Enable
  Constant26/1 -> TRCK_ID3_RX/1(In1), TRCK1_ID3_TX/1(In1)
  AND10/1 -> TRCK1_ID3_TX/Trigger
  NOT5/1 -> AND11/2
  Constant20/1 -> Equal14/2
  Constant21/1 -> Equal8/2
  Equal15/1 -> AND13/1, AND12/1
  Equal8/1 -> AND12/2, NOT6/1
  AND13/1 -> TRLS_ID4_RX/Enable
  Constant8/1 -> TRLS_ID4_RX/1(In1), TRLS_ID4_TX/1(In1)
  AND12/1 -> TRLS_ID4_TX/Trigger
  NOT6/1 -> AND13/2
  Constant22/1 -> Equal15/2
  Constant24/1 -> Equal16/2
  Equal17/1 -> AND15/1, AND14/1
  Role/1 -> Backup system/1(role), Equal16/1, Equal8/1, Equal7/1, Equal5/1, Equal3/1, Equal12/1, Equal11/1, Equal10/1
  Equal16/1 -> AND14/2, NOT7/1
  AND15/1 -> TRLS_ID5_RX/Enable
  Constant18/1 -> TRLS_ID5_RX/1(In1), TRLS_ID5_TX/1(In1)
  AND14/1 -> TRLS_ID5_TX/Trigger
  NOT7/1 -> AND15/2
  Constant25/1 -> Equal17/2
  Slot/1 -> Equal13/1, Equal6/1, Equal14/1, Equal15/1, Equal17/1, Equal2/1, Equal1/1, Equal/1
  Constant13/1 -> Equal11/2
  Equal11/1 -> OR/1
  OR/1 -> AND2/2, NOT1/1
  Backup system/1(Out1) -> OR2/2, OR1/2, OR/2
  Equal10/1 -> OR1/1
  OR1/1 -> NOT/1, AND/2
  Equal12/1 -> OR2/1
  OR2/1 -> NOT2/1, AND4/2

== system HANcoder_E407_TTA_CombineModel/HANcoder STM32 Target - E407-STM32 algorithm/Output Compare Init ==
  S-Function : S-Function  FunctionName=sfcn_timeout_init  SFunctionDeploymentMode=off  EnableBusSupport=off
  Term1 : Terminator
  wires:
  S-Function/1 -> Term1/1

== system HANcoder_E407_TTA_CombineModel/HANcoder STM32 Target - E407-STM32 algorithm/Role assignment ==
  In1 : Inport
  AND : Logic  IconShape=distinctive  AllPortsSameDT=off  OutDataTypeStr=boolean
  AND1 : Logic  IconShape=distinctive  AllPortsSameDT=off  OutDataTypeStr=boolean
  Constant : Constant  Value=ClockOn
  Constant1 : Constant  OutDataTypeStr=uint8
  Constant4 : Constant  OutDataTypeStr=uint8
  Data Store Memory : DataStoreMemory  DataStoreName=slaveClockOn  WriteAfterWriteMsg=warning  ShowAdditionalParam=off  OutDataTypeStr=boolean
  Data Store Read : DataStoreRead  DataStoreName=slaveClockOn  IndexOptions=Index vector (dialog)  Indices=1  OutputSizes=1
  Data Store Read2 : DataStoreRead  DataStoreName=slaveClockOn  IndexOptions=Index vector (dialog)  Indices=1  OutputSizes=1
  GreaterThan : RelationalOperator  Operator=>  OutDataTypeStr=boolean  RndMeth=Simplest  InputSameDT=off
  Less Than : RelationalOperator  Operator===  OutDataTypeStr=boolean  RndMeth=Simplest  InputSameDT=off
  NOT : Logic  Operator=NOT  IconShape=distinctive  AllPortsSameDT=off  OutDataTypeStr=boolean
  OR : Logic  Operator=OR  IconShape=distinctive  AllPortsSameDT=off  OutDataTypeStr=boolean
  Subsystem : Subsystem
  Subsystem2 : Subsystem
  Clock_State : Outport
  wires:
  Constant/1 -> AND/1
  AND/1 -> OR/1, Subsystem/Trigger
  Less Than/1 -> AND/2
  In1/1 -> Less Than/1, GreaterThan/1
  Constant4/1 -> Less Than/2
  Constant1/1 -> GreaterThan/2
  GreaterThan/1 -> AND1/1
  Data Store Read/1 -> NOT/1
  NOT/1 -> AND1/2
  AND1/1 -> Subsystem2/Enable
  Data Store Read2/1 -> OR/2
  OR/1 -> Clock_State/1

== system HANcoder_E407_TTA_CombineModel/HANcoder STM32 Target - E407-STM32 algorithm/Setting ID ==
  Action Port : ActionPort  ActionPortLabel=if(u1 == 0)
  Add : Sum  Inputs=+++  AccumDataTypeStr=uint8
  Constant1 : Constant  OutDataTypeStr=uint8
  Constant4 : Constant  Value=2  OutDataTypeStr=uint8
  Constant6 : Constant  Value=4  OutDataTypeStr=uint8
  Digital Input : HANcoder_STM32_Target/STM32-E407/Digital Inputs/Digital Input  Tag=HANcoder_TARGET_STM32_E407  pinID=CON4 - D8 - 5V Tolerant  config=Pulldown  tsamp=-1
      settings: SourceProductName=HANcoder STM32 Target
  Digital Input1 : HANcoder_STM32_Target/STM32-E407/Digital Inputs/Digital Input  Tag=HANcoder_TARGET_STM32_E407  pinID=CON4 - D9 - 5V Tolerant  config=Pulldown  tsamp=-1
      settings: SourceProductName=HANcoder STM32 Target
  Digital Input2 : HANcoder_STM32_Target/STM32-E407/Digital Inputs/Digital Input  Tag=HANcoder_TARGET_STM32_E407  pinID=CON4 - D10  config=Pulldown  tsamp=-1
      settings: SourceProductName=HANcoder STM32 Target
  Multiply : Product  OutDataTypeStr=uint8
  Multiply1 : Product  OutDataTypeStr=uint8
  Multiply2 : Product  OutDataTypeStr=uint8
  Output : Outport
  wires:
  Constant4/1 -> Multiply1/1
  Multiply/1 -> Add/1
  Constant1/1 -> Multiply/1
  Multiply1/1 -> Add/2
  Multiply2/1 -> Add/3
  Constant6/1 -> Multiply2/1
  Digital Input/1 -> Multiply/2
  Digital Input1/1 -> Multiply1/2
  Digital Input2/1 -> Multiply2/2
  Add/1 -> Output/1

== system HANcoder_E407_TTA_CombineModel/HANcoder STM32 Target - E407-STM32 algorithm/Spars Slots ==
  In1 : Inport
  Constant27 : Constant  Value=10
  Constant4 : Constant  Value=5
  Equal19 : RelationalOperator  Operator===  OutDataTypeStr=boolean  RndMeth=Simplest  InputSameDT=off
  Equal4 : RelationalOperator  Operator===  OutDataTypeStr=boolean  RndMeth=Simplest  InputSameDT=off
  OR1 : Logic  Operator=OR  IconShape=distinctive  AllPortsSameDT=off  OutDataTypeStr=boolean
  Out1 : Outport
  wires:
  Equal19/1 -> OR1/2
  In1/1 -> Equal19/1, Equal4/1
  Equal4/1 -> OR1/1
  OR1/1 -> Out1/1
  Constant4/1 -> Equal4/2
  Constant27/1 -> Equal19/2

== system HANcoder_E407_TTA_CombineModel/HANcoder STM32 Target - E407-STM32 algorithm/System information ==
  note: These blocks check the free memory: stack and heap and the CPU load,
      | this way you can see whether your software demands too much of the microcontroller
  Get CPU load : HANcoder_STM32_Target/STM32-E407/System Management/Get CPU load  Tag=HANcoder_TARGET_STM32_E407  mode=Current CPU load  tsamp=-1
      settings: SourceProductName=HANcoder STM32 Target
  Get free Heap : HANcoder_STM32_Target/STM32-E407/System Management/Get free Heap  Tag=HANcoder_TARGET_STM32_E407  tsamp=-1
      settings: SourceProductName=HANcoder STM32 Target
  Get free Stack : HANcoder_STM32_Target/STM32-E407/System Management/Get free Stack  Tag=HANcoder_TARGET_STM32_E407  taskIdx=Application Control Task  tsamp=-1
      settings: SourceProductName=HANcoder STM32 Target
  Terminator : Terminator
  Terminator1 : Terminator
  Terminator2 : Terminator
  wires:
  Get CPU load/1 -> Terminator1/1  "SI_CPUload"
  Get free Stack/1 -> Terminator/1  "SI_FreeStack"
  Get free Heap/1 -> Terminator2/1  "SI_FreeHeap"

== system HANcoder_E407_TTA_CombineModel/HANcoder STM32 Target - E407-STM32 algorithm/Triggered Subsystem ==
  Action Port : ActionPort  ActionPortLabel=if(u1 <= 3)
  Add : Sum
  Cast{,1..3} (4 alike) : DataTypeConversion  SaturateOnIntegerOverflow=off  RndMeth=Floor
  Data Store Read : DataStoreRead  DataStoreName=trailer1buttonPress  IndexOptions=Index vector (dialog)  Indices=1  OutputSizes=1
  Data Store Read1 : DataStoreRead  DataStoreName=trailer2buttonPress  IndexOptions=Index vector (dialog)  Indices=1  OutputSizes=1
  Data Store Read45 : DataStoreRead  DataStoreName=PositionID5  IndexOptions=Index vector (dialog)  Indices=1  OutputSizes=1
  Data Store Read46 : DataStoreRead  DataStoreName=PositionID4  IndexOptions=Index vector (dialog)  Indices=1  OutputSizes=1
  Data Store Write12 : DataStoreWrite  DataStoreName=PositionID5  IndexOptions=Index vector (dialog)  Indices=1  OutputSizes=1
  Data Store Write13 : DataStoreWrite  DataStoreName=amountOfTrailers  IndexOptions=Index vector (dialog)  Indices=1  OutputSizes=1
  Data Store Write6 : DataStoreWrite  DataStoreName=PositionID4  IndexOptions=Index vector (dialog)  Indices=1  OutputSizes=1
  Digital Input1 : HANcoder_STM32_Target/STM32-E407/Digital Inputs/Digital Input  Tag=HANcoder_TARGET_STM32_E407  pinID=WKUP button  config=Pulldown  tsamp=-1
      settings: SourceProductName=HANcoder STM32 Target
  Saturation : Saturate  UpperLimit=1  LowerLimit=0
  Saturation1 : Saturate  UpperLimit=1  LowerLimit=0
  Subsystem : Subsystem
  wires:
  Data Store Read45/1 -> Saturation1/1
  Saturation1/1 -> Add/2
  Saturation/1 -> Add/1
  Data Store Read46/1 -> Saturation/1
  Digital Input1/1 -> Subsystem/Enable
  Subsystem/2(Position ID12) -> Cast3/1
  Subsystem/1(Position ID11) -> Cast2/1
  Add/1 -> Data Store Write13/1  "amounttrailers"
  Cast2/1 -> Data Store Write6/1  "positionID4"
  Cast3/1 -> Data Store Write12/1  "positionID5"
  Data Store Read1/1 -> Cast/1
  Data Store Read/1 -> Cast1/1
  Cast1/1 -> Subsystem/1(In1)
  Cast/1 -> Subsystem/2(In2)

== system HANcoder_E407_TTA_CombineModel/HANcoder STM32 Target - E407-STM32 algorithm/Control execution/Control Algorithm ==
  note: The gains here are to determine the angles from 0 - 60
  Kinematic output : Inport
  AND : Logic  IconShape=distinctive  AllPortsSameDT=off  OutDataTypeStr=boolean
  AND1 : Logic  IconShape=distinctive  AllPortsSameDT=off  OutDataTypeStr=boolean
  Abs : Abs  OutDataTypeStr=double  SaturateOnIntegerOverflow=off
  Add : Sum  AccumDataTypeStr=uint16
  Cast : DataTypeConversion  OutDataTypeStr=uint16  SaturateOnIntegerOverflow=off  RndMeth=Floor
  Cast1 : DataTypeConversion  OutDataTypeStr=boolean  SaturateOnIntegerOverflow=off  RndMeth=Floor
  Cast3 : DataTypeConversion  SaturateOnIntegerOverflow=off  RndMeth=Floor
  Constant : Constant  Value=controlWidth
  Constant1 : Constant  Value=0
  Data Store Read : DataStoreRead  DataStoreName=encoderPosition  IndexOptions=Index vector (dialog)  Indices=1  OutputSizes=1
  Discrete PID Controller1 : slpidlib/PID Controller  Controller=PI  Form=Parallel  TimeDomain=Discrete-time  UseExternalTs=off  SampleTime=-1  IntegratorMethod=Forward Euler  FilterMethod=Forward Euler  ControllerParametersSource=internal  P=propVal  I=intVal  UseKiTs=on  D=0.5  N=100  UseFilter=on  TunerSelectOption=Transfer Function Based (PID Tuner App)  InitialConditionSource=internal  InitialConditionForIntegrator=0  InitialConditionForFilter=0  DifferentiatorICPrevScaledInput=0  ExternalReset=none  TrackingMode=off  Kt=1  LimitOutput=on  SatLimitsSource=internal  UpperSaturationLimit=300  LowerSaturationLimit=0  LinearizeAsGain=off  AntiWindupMode=clamping  Kb=1  LimitIntegrator=on  UpperIntegratorSaturationLimit=100  LowerIntegratorSaturationLimit=0  POutMin=[]  POutMax=[]  IOutMin=[]  IOutMax=[]  DOutMin=[]  DOutMax=[]  NOutMin=[]  NOutMax=[]  SumOutMin=[]  SumOutMax=[]  SaturationOutMin=[]  SaturationOutMax=[]  PParamMin=[]  PParamMax=[]  IParamMin=[]  IParamMax=[]  DParamMin=[]  DParamMax=[]  NParamMin=[]  NParamMax=[]  KbParamMin=[]  KbParamMax=[]  KtParamMin=[]  KtParamMax=[]  KbOutMin=[]  KbOutMax=[]  KtOutMin=[]  KtOutMax=[]  IntegratorOutMin=[]  IntegratorOutMax=[]  FilterOutMin=[]  FilterOutMax=[]  SumI1OutMin=[]  SumI1OutMax=[]  SumI2OutMin=[]  SumI2OutMax=[]  SumI3OutMin=[]  SumI3OutMax=[]  SumI4OutMin=[]  SumI4OutMax=[]  SumDOutMin=[]  SumDOutMax=[]  DifferentiatorOutMin=[]  DifferentiatorOutMax=[]  FilterDiffOutCoefMin=[]  FilterDiffOutCoefMax=[]  ReciprocalOutMin=[]  ReciprocalOutMax=[]  SumDenOutMin=[]  SumDenOutMax=[]  SumNumOutMin=[]  SumNumOutMax=[]  DivideOutMin=[]  DivideOutMax=[]  UdiffTsProdOutMin=[]  UdiffTsProdOutMax=[]  NTsProdOutMin=[]  NTsProdOutMax=[]  UintegralTsProdOutMin=[]  UintegralTsProdOutMax=[]  UngainTsProdOutMin=[]  UngainTsProdOutMax=[]  ClampingZeroOutDataTypeStr=Inherit: Inherit via back propagation  ClampingZeroOutMin=[]  ClampingZeroOutMax=[]  FilterDenConstantOutDataTypeStr=Inherit: Inherit via back propagation  FilterDenConstantOutMin=[]  FilterDenConstantOutMax=[]  PCopyOutDataTypeStr=Inherit: Inherit via back propagation  PCopyOutMin=[]  PCopyOutMax=[]  NCopyOutDataTypeStr=Inherit: Inherit via back propagation  NCopyOutMin=[]  NCopyOutMax=[]  IntegratorContinuousStateAttributes=''  IntegratorStateMustResolveToSignalObject=off  IntegratorRTWStateStorageClass=Auto  FilterContinuousStateAttributes=''  FilterStateMustResolveToSignalObject=off  FilterRTWStateStorageClass=Auto  ParallelPVariant=InternalParameters  IdealPVariant=Disabled  IVariant=InternalParameters  DVariant=Disabled  IntegratorVariant=Discrete  SatVariant=Enabled  AWVariant=DiscClampingParallel  PCopyVariant=Disabled  TRVariant=Disabled  FdbkBlocksVariant=Forward  IdealPFdbkVariant=Disabled  SatFdbkVariant=Disabled  DerivativeFilterVariant=Disabled  NVariant=Disabled  NCopyVariant=Disabled_SignalSpec  FilterICVariant=Disabled  IntegratorICVariant=InternalICs  ExternalResetVariant=Disabled  TRSumVariant=Passthrough  SumFdbkVariant=Disabled  SumVariant=Sum_PI  TsampFilterVariant=InternalTs  TsampNgainVariant=Passthrough  TsampIntegralVariant=Passthrough  ExternalSaturationOutDataTypeStr=Inherit: Same as second input
  Gain1 : Gain  Gain=1/10  OutDataTypeStr=double
  Gain2 : Gain  Gain=45.6
  GreaterThan : RelationalOperator  Operator=>  OutDataTypeStr=boolean  RndMeth=Simplest  InputSameDT=off
  GreaterThan1 : RelationalOperator  Operator=>  OutDataTypeStr=boolean  RndMeth=Simplest  InputSameDT=off
  Motor dead zone : Constant  Value=500  OutDataTypeStr=uint16
  NOT : Logic  Operator=NOT  IconShape=distinctive  AllPortsSameDT=off  OutDataTypeStr=boolean
  Round : Rounding
  Round1 : Rounding
  Sum : Sum  Inputs=+-
  Motor speed : Outport
  CW direction : Outport  Port=2
  CCW direction : Outport  Port=3
  wires:
  Motor dead zone/1 -> Add/1
  Sum/1 -> GreaterThan/1, Abs/1  "control"
  Abs/1 -> Discrete PID Controller1/1, GreaterThan1/1
  GreaterThan/1 -> Cast1/1
  Cast1/1 -> AND/2, NOT/1  "cw"
  Add/1 -> Motor speed/1  "mospeed"
  Constant1/1 -> GreaterThan/2
  Gain1/1 -> Round1/1  "position"
  Discrete PID Controller1/1 -> Cast/1
  Gain2/1 -> Round/1  "steering"
  Round/1 -> Sum/1
  Round1/1 -> Sum/2
  Data Store Read/1 -> Gain1/1
  Cast/1 -> Add/2
  GreaterThan1/1 -> AND/1, AND1/1
  Constant/1 -> GreaterThan1/2
  AND/1 -> CW direction/1
  NOT/1 -> AND1/2  "ccw"
  AND1/1 -> CCW direction/1
  Cast3/1 -> Gain2/1
  Kinematic output/1 -> Cast3/1

== system HANcoder_E407_TTA_CombineModel/HANcoder STM32 Target - E407-STM32 algorithm/Control execution/Kinematic Algorithm ==
  note: Here the algorithm can be placed. No hardware dependent blocks should be used here.
  note: Tractor angle is probably a constant or 0
  note: DeltaC is taken from the potentiometer
  note: This is just an angle, it has to be transformed to a raw values for computation
  note: Trailer angle values have to be assigned
      |  from reading the messages
  DeltaC : Inport
  V2 : Inport  Port=2
  YawTractorAngle : Inport  Port=3
  YawTrailer1Angle : Inport  Port=4
  YawTrailer2Angle : Inport  Port=5
  1st trailer local velocity : Subsystem
  1st trailer yew rate : Subsystem
  2nd Trailer yaw rate : Subsystem
  RearAxleToHitch : Constant  Value=L0b
  Steer angle at steer axle : Subsystem
  Sum1 : Sum  Inputs=-+
  Sum2 : Sum  Inputs=-+
  Tractor local velocity : Subsystem
  Tractor yaw rate : Subsystem
  TractorWheelbase : Constant  Value=L0F
  TrailUnitWheelbase : Constant  Value=L1F
  Delta12K : Outport
  wires:
  Tractor local velocity/1(V0) -> Steer angle at steer axle/1(V0)
  RearAxleToHitch/1 -> Tractor yaw rate/5(L0b), 1st trailer yew rate/4(L0b)
  2nd Trailer yaw rate/1(ThetaDot2) -> 1st trailer local velocity/4(ThetaDot2), 1st trailer yew rate/1(ThetaDot2)
  Sum2/1 -> 1st trailer local velocity/1(Gamma2), 1st trailer yew rate/5(Gamma2)  "Gamma2"
  Sum1/1 -> Tractor yaw rate/1(Gamma1), Tractor local velocity/4(Gamma1)  "Gamma1"
  1st trailer yew rate/1(ThetaDot1) -> Tractor yaw rate/2(ThetaDot1), Tractor local velocity/1(ThetaDot1)
  YawTrailer1Angle/1 -> Sum1/1, Sum2/2
  V2/1 -> 1st trailer yew rate/2(V2), 1st trailer local velocity/2(V2), 2nd Trailer yaw rate/2(V2)
  YawTrailer2Angle/1 -> Sum2/1
  TrailUnitWheelbase/1 -> Tractor yaw rate/4(L1F), Tractor local velocity/3(L1F), 1st trailer local velocity/3(L1F), 1st trailer yew rate/3(L1F), 2nd Trailer yaw rate/3(L1F)
  Steer angle at steer axle/1(Delta12K) -> Delta12K/1
  1st trailer local velocity/1(V1) -> Tractor yaw rate/3(V1), Tractor local velocity/2(V1)
  DeltaC/1 -> 2nd Trailer yaw rate/1(Deltac)
  Tractor yaw rate/1(ThetaDot0) -> Steer angle at steer axle/2(L0f)
  TractorWheelbase/1 -> Steer angle at steer axle/3(ThetaDot0)
  YawTractorAngle/1 -> Sum1/2
